simulink model "Sim_PTSMC"  (R2025b)
settings: Solver=ode4  StartTime=0.0  StopTime=10  FixedStep=0.001  RelTol=1e-3  EnableMultiTasking=on
settings Model: ExtModeTrigMode=oneshot  ExtModeArmWhenConnect=off  Creator=J  LastModifiedBy=J
settings DataIOCC: SaveFormat=Array  SignalLoggingSaveFormat=ModelDataLogs  ReturnWorkspaceOutputs=off  SignalLoggingName=sigsOut
settings OptimizationCC: BooleanDataType=off  ReuseModelBlockBuffer=off
settings DebuggingCC: SaveWithParameterizedLinksMsg=none  UnderspecifiedInitializationDetection=Classic  MergeDetectMultiDrivingBlocksExec=none  SignalResolutionControl=TryResolveAllWithWarning  MultiTaskDSMMsg=warning  MultiTaskCondExecSysMsg=none  UnconnectedInputMsg=warning  UnconnectedOutputMsg=warning  UnconnectedLineMsg=warning
settings HardwareCC: ProdBitPerPointer=32.0  ProdBitPerSizeT=32.0  ProdBitPerPtrDiffT=32.0  ProdLargestAtomicFloat=None  ProdIntDivRoundTo=Undefined  ProdEndianess=Unspecified  ProdWordSize=32.0  ProdHWDeviceType=32-bit Generic  TargetUnknown=on
settings ModelReferenceCC: PropagateSignalLabelsOutOfModel=off
settings RTWCC: GPUComputeCapability=3.5
settings GRTTargetCC: CombineOutputUpdateFcns=off  GRTInterface=on
settings ConfigComp: CovMetricSettings=dw  CovSaveCumulativeToWorkspaceVar=on  CovSaveSingleToWorkspaceVar=on
settings SimscapeCC: SimscapeLogDataHistory=5000  SimscapeLogDecimation=1

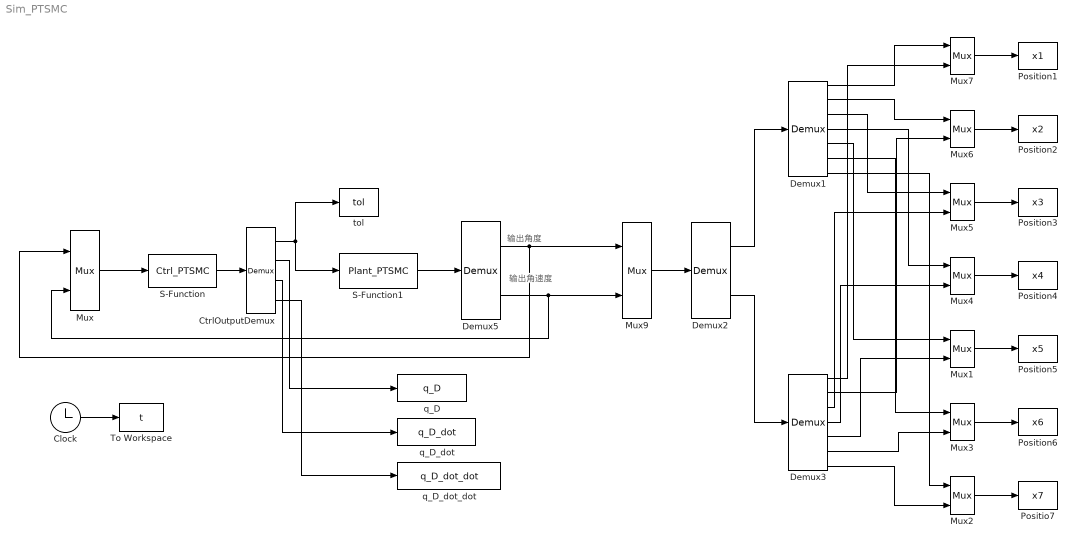
== system Sim_PTSMC ==
  note: 输出角度
  note: 输出角速度
  Clock : Clock
  CtrlOutputDemux : Demux
      settings: DisplayOption=none
  Demux1 : Demux  Outputs=7
      settings: DisplayOption=none
  Demux2 : Demux  Outputs=2
      settings: DisplayOption=none
  Demux3 : Demux  Outputs=7
      settings: DisplayOption=none
  Demux5 : Demux  Outputs=2
      settings: DisplayOption=none
  Mux{,1..7,9} (9 alike) : Mux  Inputs=2
  Positio7 : ToWorkspace  VariableName=x7  SampleTime=-1
  Position1 : ToWorkspace  VariableName=x1  SampleTime=-1
  Position2 : ToWorkspace  VariableName=x2  SampleTime=-1
  Position3 : ToWorkspace  VariableName=x3  SampleTime=-1
  Position4 : ToWorkspace  VariableName=x4  SampleTime=-1
  Position5 : ToWorkspace  VariableName=x5  SampleTime=-1
  Position6 : ToWorkspace  VariableName=x6  SampleTime=-1
  S-Function : S-Function  FunctionName=Ctrl_PTSMC  SFunctionDeploymentMode=off  EnableBusSupport=off
  S-Function1 : S-Function  FunctionName=Plant_PTSMC  SFunctionDeploymentMode=off  EnableBusSupport=off
  To Workspace : ToWorkspace  VariableName=t  SampleTime=-1
  q_D : ToWorkspace  VariableName=q_D  SampleTime=-1
  q_D_dot : ToWorkspace  VariableName=q_D_dot  SampleTime=-1
  q_D_dot_dot : ToWorkspace  VariableName=q_D_dot_dot  SampleTime=-1
  tol : ToWorkspace  VariableName=tol  SampleTime=-1
  wires:
  Mux/1 -> S-Function/1
  Mux2/1 -> Positio7/1
  Mux3/1 -> Position6/1
  Clock/1 -> To Workspace/1
  Mux1/1 -> Position5/1
  Mux4/1 -> Position4/1
  Mux5/1 -> Position3/1
  Mux6/1 -> Position2/1
  Mux7/1 -> Position1/1
  S-Function/1 -> CtrlOutputDemux/1
  CtrlOutputDemux/1 -> tol/1, S-Function1/1
  CtrlOutputDemux/2 -> q_D/1
  CtrlOutputDemux/3 -> q_D_dot/1
  CtrlOutputDemux/4 -> q_D_dot_dot/1
  Mux9/1 -> Demux2/1
  S-Function1/1 -> Demux5/1
  Demux5/1 -> Mux/1, Mux9/1
  Demux5/2 -> Mux9/2, Mux/2
  Demux2/1 -> Demux1/1
  Demux2/2 -> Demux3/1
  Demux1/1 -> Mux7/1
  Demux1/2 -> Mux6/1
  Demux1/3 -> Mux5/1
  Demux1/4 -> Mux4/1
  Demux1/5 -> Mux1/1
  Demux1/6 -> Mux3/1
  Demux1/7 -> Mux2/1
  Demux3/1 -> Mux7/2
  Demux3/2 -> Mux6/2
  Demux3/3 -> Mux5/2
  Demux3/4 -> Mux4/2
  Demux3/5 -> Mux1/2
  Demux3/6 -> Mux3/2
  Demux3/7 -> Mux2/2
